simulink model "Motor"  (R2018b)
settings: Solver=VariableStepAuto  StartTime=0.0  StopTime=10.0  RelTol=1e-3
libraries: fl_lib x7, elec_lib x3, nesl_utility x2
settings Model: Creator=Cristian  LastModifiedBy=Cristian

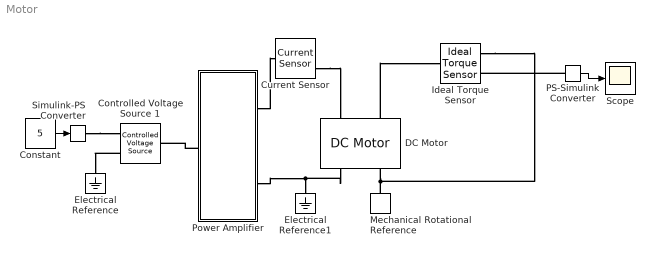
== system Motor ==
  Constant : Constant  Value=5
  Controlled Voltage Source 1 : fl_lib/Electrical/Electrical Sources/Controlled Voltage Source
  Current Sensor : fl_lib/Electrical/Electrical Sensors/Current Sensor
  DC Motor : elec_lib/Actuators & Drivers/Rotational Actuators/DC Motor  parameterization=1  Ra=3.9 Ohm  La=12e-6 H  emf_or_torque=1  Kv=0.072e-3 V/rpm  Ki=6.876e-4 N*m/A  T_stall=0.24e-3 N*m  w_max=19100 rpm  w_rated=15000 rpm  P_rated=0.08 W  V_rated=1.5 V  J=0.01 g*cm^2  lam_param=1  lam=0 N*m/(rad/s)  i_noload=0 A  V_i_noload=1.5 V  speed0=0 rpm  alpha=3.93e-3 1/K  Tmeas=25 degC  thermal_mass=100 J/K  initial_temperature=25 degC
  Electrical Reference : fl_lib/Electrical/Electrical Elements/Electrical Reference
  Electrical Reference1 : fl_lib/Electrical/Electrical Elements/Electrical Reference
  Ideal Torque Sensor : fl_lib/Mechanical/Mechanical Sensors/Ideal Torque Sensor
  Mechanical Rotational Reference : fl_lib/Mechanical/Rotational Elements/Mechanical Rotational Reference
  PS-Simulink Converter : nesl_utility/PS-Simulink Converter  PhysicalDomain=network_engine_domain  SubClassName=ps_output  LeftPortType=input  RightPortType=output  PseudoPeriodic=off  Frequencies=[]  Unit=1  AffineConversion=off
  Power Amplifier : Subsystem
  Scope : Scope
  Simulink-PS Converter : nesl_utility/Simulink-PS Converter  PhysicalDomain=network_engine_domain  SubClassName=ps_input  LeftPortType=input  RightPortType=output  PseudoPeriodic=off  Frequencies=[]  NoiseDistribution=none  NoiseParameters=[]  Unit=1  AffineConversion=off  FilteringAndDerivatives=provide  SimscapeFilterOrder=1  InputFilterTimeConstant=0.001  UdotUserProvided=0
  wires:
  PS-Simulink Converter/1 -> Scope/1
  Constant/1 -> Simulink-PS Converter/1
  connections:
  Electrical Reference1/LConn1 -- Power Amplifier/RConn2 -- DC Motor/RConn1
  Mechanical Rotational Reference/LConn1 -- Ideal Torque Sensor/RConn1 -- DC Motor/RConn2
  Power Amplifier/RConn1 -- Current Sensor/LConn1
  Power Amplifier/LConn1 -- Controlled Voltage Source 1/LConn1
  Controlled Voltage Source 1/RConn2 -- Electrical Reference/LConn1
  Simulink-PS Converter/RConn1 -- Controlled Voltage Source 1/RConn1
  DC Motor/LConn2 -- Ideal Torque Sensor/LConn1
  Current Sensor/RConn2 -- DC Motor/LConn1
  PS-Simulink Converter/LConn1 -- Ideal Torque Sensor/RConn2

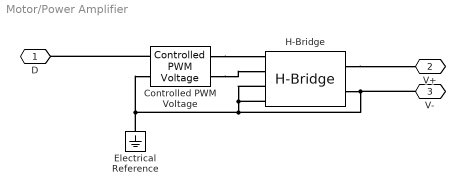
== system Motor/Power Amplifier ==
  Controlled PWM Voltage : elec_lib/Actuators & Drivers/Drivers/Controlled PWM Voltage  F=1000 Hz  TD=0 s  pulse_width_offset=0 s  pulse_min=0 s  Vmin=0 V  Vmax=5 V  Vm=5 V  pwm_or_av=2  event_type=1  sample_time=1e-6 s  u_min=0  u_max=1
      settings: SourceProductName=Simscape Electronics  SourceProductBaseCode=SN
  Electrical Reference : fl_lib/Electrical/Electrical Elements/Electrical Reference
  H-Bridge : elec_lib/Actuators & Drivers/Drivers/H-Bridge  Venable=2.5 V  Vmax=5.0 V  Vreverse=2.5 V  Vbrake=2.5 V  Vm=12 V  pwm_or_av=1  discontinuous=0  freewheeling_mode=1  freewheeling_mode_disc=1  Ron=0.1 Ohm  Don=0.05 Ohm  Rload=10 Ohm  Lload=1e-5 H  F=10 kHz  thermal_mass=100 J/K  initial_temperature=298.15 K  Ron2=0.1 Ohm  Don2=0.05 Ohm  Tmeas=298.15 K  Tmeas2=398.15 K
      settings: SourceProductName=Simscape Electronics  SourceProductBaseCode=SN
  D : PMIOPort  Side=Left
  V+ : PMIOPort  Port=2  Side=Right
  V- : PMIOPort  Port=3  Side=Right
  connections:
  Controlled PWM Voltage/RConn2 -- H-Bridge/LConn2
  Controlled PWM Voltage/RConn1 -- H-Bridge/LConn1
  Controlled PWM Voltage/LConn2 -- Electrical Reference/LConn1 -- H-Bridge/LConn4 -- H-Bridge/LConn3 -- H-Bridge/RConn2 -- V-/RConn1
  Controlled PWM Voltage/LConn1 -- D/RConn1
  H-Bridge/RConn1 -- V+/RConn1
